simulink model "NewModelAtomicTest"  (R2017a)
settings: Solver=VariableStepAuto  StartTime=0.0  StopTime=.2  RelTol=1e-3
settings Model: Creator=erich  LastModifiedBy=erich

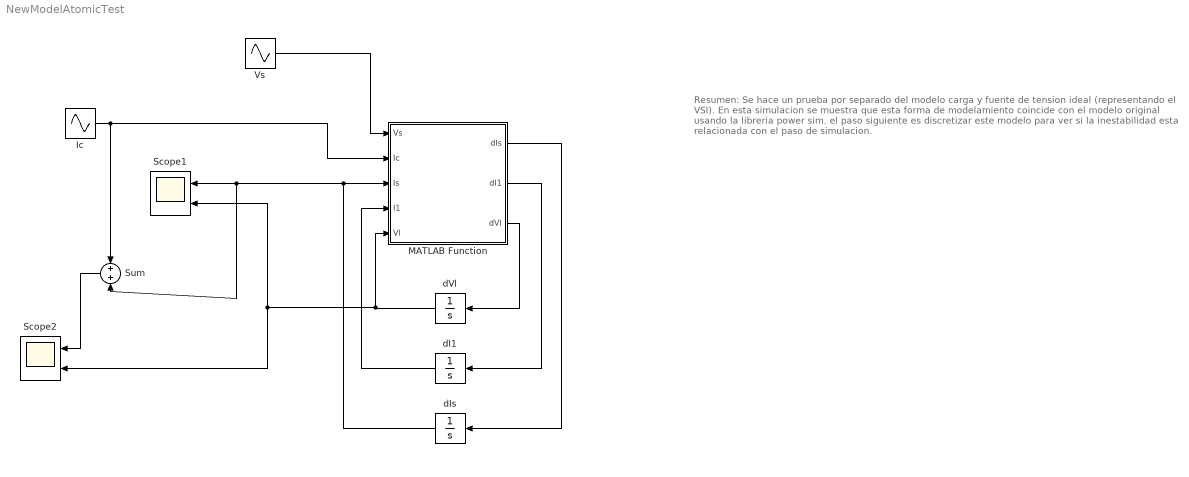
== system NewModelAtomicTest ==
  note: Resumen:
      | Se hace un prueba por separado del modelo
      | carga y fuente de tension ideal (representando el VSI).
      | En esta simulacion se muestra que esta forma de modelamiento
      | coincide con el modelo original usando la libreria power sim.
      |
      | el paso siguiente es discretizar este modelo para ver si la inestabilidad
      | esta relacionada con el paso de simulacion.
  Ic : Sin  Amplitude=50  Frequency=2*pi*60  Phase=-2*pi/5  SampleTime=0
  MATLAB Function : MATLAB Function  TreatAsAtomicUnit=on
  Scope1 : Scope  NumInputPorts=2
  Scope2 : Scope  NumInputPorts=2
  Sum : Sum  Inputs=+|+
  Vs : Sin  Amplitude=170  Frequency=2*pi*60  SampleTime=0
  dI1 : Integrator
  dIs : Integrator
  dVl : Integrator
  wires:
  MATLAB Function/3(dVl) -> dVl/1
  dVl/1 -> Scope1/2, Scope2/2, MATLAB Function/5(Vl)
  MATLAB Function/2(dI1) -> dI1/1
  dI1/1 -> MATLAB Function/4(I1)
  MATLAB Function/1(dIs) -> dIs/1
  dIs/1 -> Sum/2, Scope1/1, MATLAB Function/3(Is)
  Vs/1 -> MATLAB Function/1(Vs)
  Ic/1 -> Sum/1, MATLAB Function/2(Ic)
  Sum/1 -> Scope2/1

== matlab function NewModelAtomicTest/MATLAB Function ==
  data: Vs input; dIs output; Ic input; Is input; I1 input; Vl input; dI1 output; dVl output
function [dIs, dI1, dVl] = fcn(Vs, Ic, Is, I1, Vl)

% parametros
rs = 1e-3; % parte resistiva impedancia de linea
Ls = 1e-6; % parte inductiva impedancia de linea

% valores de los componentes de la carga.
Cl = 2000e-6;
Ll = 5.2;
rl = 10; 
Rl = 10;

dIs = ((Vs-Vl)-Is*rs)/Ls;

dI1 = (Vl - I1*rl)/Ll;

dVl = ( (Ic+Is) -I1 -(Vl/Rl) )/Cl;
